simulink library "LIB_TF_G_12_StepControl"  (Simulink 8.6)
settings: Solver=ode45  StartTime=0.0  StopTime=10.0  RelTol=1e-3
PreLoadFcn:
  | if exist('tl_preloadfcn','file'), tl_preloadfcn(gcs,402); end
PostLoadFcn:
  | if exist('tl_postloadfcn','file'), tl_postloadfcn(gcs,402); end
undefined symbols (not defined in the file): ddv, u2, u3
libraries: tllib x4, LIB_TF_G_12_StepControl x1
(part 3 of 7)

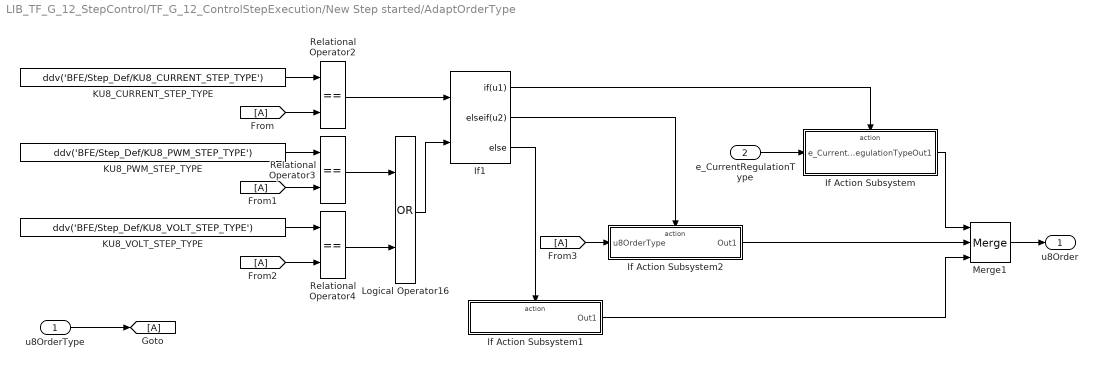
== system LIB_TF_G_12_StepControl/TF_G_12_ControlStepExecution/New Step started/AdaptOrderType ==
  u8OrderType : Inport  RequirementInfo={} %GIDa_d0932c2d_2946_4ca8_ae3e_f63aac2e144a
  e_CurrentRegulationType : Inport  RequirementInfo={} %GIDa_1019e4f9_7aa8_470e_93c0_bc7d62933626  Port=2
  If Action Subsystem : Subsystem  RequirementInfo={} %GIDa_16aa67de_e04f_4aef_8846_7bc2339db7f1  TreatAsAtomicUnit=on
  If Action Subsystem1 : Subsystem  RequirementInfo={} %GIDa_efde54be_58e1_48f4_984b_1a55cd541708  TreatAsAtomicUnit=on
  If Action Subsystem2 : Subsystem  RequirementInfo={} %GIDa_7e05d702_bec6_4133_89e3_7df1c2d817b3  TreatAsAtomicUnit=on
  If1 : If  RequirementInfo={} %GIDa_230b83ff_c373_44fd_bf0d_fc368a5a2e7f  NumInputs=2  IfExpression=u1  ElseIfExpressions=u2
  KU8_CURRENT_STEP_TYPE : Constant  RequirementInfo={} %GIDa_98379601_80fc_49bf_9245_1ac9e089f011  Value=ddv('BFE/Step_Def/KU8_CURRENT_STEP_TYPE')  OutDataTypeStr=uint8  mask(TL_Constant){data={'output',{'variable','BFE/Step_Def/KU8_CURRENT_STEP_TYPE'},'date',735951.66797598382}}
      settings: CopyFcn=if exist('tl_reset_reviewflag','file')==2,tl_reset_reviewflag(gcbh);end  DeleteFcn=if exist('delete_tlblock','file')==2,delete_tlblock(gcbh);end  NameChangeFcn=if exist('rename_tlblock','file')==2,rename_tlblock(gcbh);end  OpenFcn=if exist('tl_open_blockdlg','file')==2,tl_open_blockdlg(gcbh);else,open_system(gcbh,'parameter');end
      mask Help: eval(['if exist(''tl_online_help'',''file'') == 2, tl_online_help(''Topic'',''TL_Constant''),else, web([''jar:file:///'',matlabroot,''/help/toolbox/simulink/help.jar!/slref/' lower(get_param(gcbh,'Blocktype')) '.html''], ''-helpbrowser''),end'])
      mask Display: plot([-0.05, 1.05, NaN, -0.05, 1.05],[.01, .01, NaN, .99, .99])
  KU8_PWM_STEP_TYPE : Constant  RequirementInfo={} %GIDa_29bcd219_c5cc_40dc_ab00_ad3704692ecd  Value=ddv('BFE/Step_Def/KU8_PWM_STEP_TYPE')  OutDataTypeStr=uint8  mask(TL_Constant){data={'output',{'variable','BFE/Step_Def/KU8_PWM_STEP_TYPE'},'date',735951.66797560186}}
      settings: CopyFcn=if exist('tl_reset_reviewflag','file')==2,tl_reset_reviewflag(gcbh);end  DeleteFcn=if exist('delete_tlblock','file')==2,delete_tlblock(gcbh);end  NameChangeFcn=if exist('rename_tlblock','file')==2,rename_tlblock(gcbh);end  OpenFcn=if exist('tl_open_blockdlg','file')==2,tl_open_blockdlg(gcbh);else,open_system(gcbh,'parameter');end
      mask Help: eval(['if exist(''tl_online_help'',''file'') == 2, tl_online_help(''Topic'',''TL_Constant''),else, web([''jar:file:///'',matlabroot,''/help/toolbox/simulink/help.jar!/slref/' lower(get_param(gcbh,'Blocktype')) '.html''], ''-helpbrowser''),end'])
      mask Display: plot([-0.05, 1.05, NaN, -0.05, 1.05],[.01, .01, NaN, .99, .99])
  KU8_VOLT_STEP_TYPE : Constant  RequirementInfo={} %GIDa_f802c029_4a46_4d43_a78a_2d66bfbde5dc  Value=ddv('BFE/Step_Def/KU8_VOLT_STEP_TYPE')  OutDataTypeStr=uint8  mask(TL_Constant){data={'output',{'variable','BFE/Step_Def/KU8_VOLT_STEP_TYPE'},'date',735951.6679752199}}
      settings: CopyFcn=if exist('tl_reset_reviewflag','file')==2,tl_reset_reviewflag(gcbh);end  DeleteFcn=if exist('delete_tlblock','file')==2,delete_tlblock(gcbh);end  NameChangeFcn=if exist('rename_tlblock','file')==2,rename_tlblock(gcbh);end  OpenFcn=if exist('tl_open_blockdlg','file')==2,tl_open_blockdlg(gcbh);else,open_system(gcbh,'parameter');end
      mask Help: eval(['if exist(''tl_online_help'',''file'') == 2, tl_online_help(''Topic'',''TL_Constant''),else, web([''jar:file:///'',matlabroot,''/help/toolbox/simulink/help.jar!/slref/' lower(get_param(gcbh,'Blocktype')) '.html''], ''-helpbrowser''),end'])
      mask Display: plot([-0.05, 1.05, NaN, -0.05, 1.05],[.01, .01, NaN, .99, .99])
  Logical Operator16 : Logic  RequirementInfo={} %GIDa_b0b2f49c_87b5_4b72_83bb_2ee36afe3fae  Operator=OR  AllPortsSameDT=off  OutDataTypeStr=boolean  mask(TL_LogicalOperator){data={'date',735951.66797486111}}
      settings: DeleteFcn=if exist('delete_tlblock','file')==2,delete_tlblock(gcbh);end  NameChangeFcn=if exist('rename_tlblock','file')==2,rename_tlblock(gcbh);end  OpenFcn=if exist('tl_open_blockdlg','file')==2,tl_open_blockdlg(gcbh);else,open_system(gcbh,'parameter');end
      mask Help: eval(['if exist(''tl_online_help'',''file'') == 2, tl_online_help(''Topic'',''TL_LogicalOperator''),else, web([''jar:file:///'',matlabroot,''/help/toolbox/simulink/help.jar!/slref/' lower(get_param(gcbh,'Blocktype')) '.html''], ''-helpbrowser''),end'])
      mask Display: plot([-0.05, 1.05, NaN, -0.05, 1.05],[.01, .01, NaN, .99, .99])
  Merge1 : Merge  RequirementInfo={} %GIDa_c83b2496_f2b0_4692_be7f_77f82a802315  Inputs=3  InitialOutput=0  mask(TL_Merge){data={'output',{'name','u8NewRawOrderType'},'date',735951.66797458334}}
      settings: CopyFcn=if exist('tl_reset_reviewflag','file')==2,tl_reset_reviewflag(gcbh);end  DeleteFcn=if exist('delete_tlblock','file')==2,delete_tlblock(gcbh);end  NameChangeFcn=if exist('rename_tlblock','file')==2,rename_tlblock(gcbh);end  OpenFcn=if exist('tl_open_blockdlg','file')==2,tl_open_blockdlg(gcbh);else,open_system(gcbh,'parameter');end
      mask Help: eval(['if exist(''tl_online_help'',''file'') == 2, tl_online_help(''Topic'',''TL_Merge''),else, web([''jar:file:///'',matlabroot,''/help/toolbox/simulink/help.jar!/slref/' lower(get_param(gcbh,'Blocktype')) '.html''], ''-helpbrowser''),end'])
      mask Display: plot([-0.05, 1.05, NaN, -0.05, 1.05],[.01, .01, NaN, .99, .99])
  Relational Operator2 : RelationalOperator  RequirementInfo={} %GIDa_18ac9ebf_a7ed_4eb9_a4e9_7db870fd7569  Operator===  OutDataTypeStr=boolean  mask(TL_RelationalOperator){data={'date',735951.66797421291}}
      settings: DeleteFcn=if exist('delete_tlblock','file')==2,delete_tlblock(gcbh);end  NameChangeFcn=if exist('rename_tlblock','file')==2,rename_tlblock(gcbh);end  OpenFcn=if exist('tl_open_blockdlg','file')==2,tl_open_blockdlg(gcbh);else,open_system(gcbh,'parameter');end
      mask Help: eval(['if exist(''tl_online_help'',''file'') == 2, tl_online_help(''Topic'',''TL_RelationalOperator''),else, web([''jar:file:///'',matlabroot,''/help/toolbox/simulink/help.jar!/slref/' lower(get_param(gcbh,'Blocktype')) '.html''], ''-helpbrowser''),end'])
      mask Display: plot([-0.05, 1.05, NaN, -0.05, 1.05],[.01, .01, NaN, .99, .99])
  Relational Operator3 : RelationalOperator  RequirementInfo={} %GIDa_1f07f267_5fe9_402f_8d87_9ef376af47f7  Operator===  OutDataTypeStr=boolean  mask(TL_RelationalOperator){data={'date',735951.66797396995}}
      settings: DeleteFcn=if exist('delete_tlblock','file')==2,delete_tlblock(gcbh);end  NameChangeFcn=if exist('rename_tlblock','file')==2,rename_tlblock(gcbh);end  OpenFcn=if exist('tl_open_blockdlg','file')==2,tl_open_blockdlg(gcbh);else,open_system(gcbh,'parameter');end
      mask Help: eval(['if exist(''tl_online_help'',''file'') == 2, tl_online_help(''Topic'',''TL_RelationalOperator''),else, web([''jar:file:///'',matlabroot,''/help/toolbox/simulink/help.jar!/slref/' lower(get_param(gcbh,'Blocktype')) '.html''], ''-helpbrowser''),end'])
      mask Display: plot([-0.05, 1.05, NaN, -0.05, 1.05],[.01, .01, NaN, .99, .99])
  Relational Operator4 : RelationalOperator  RequirementInfo={} %GIDa_fd8addad_e037_4a75_aa53_445cbc8f9875  Operator===  OutDataTypeStr=boolean  mask(TL_RelationalOperator){data={'date',735951.66797372687}}
      settings: DeleteFcn=if exist('delete_tlblock','file')==2,delete_tlblock(gcbh);end  NameChangeFcn=if exist('rename_tlblock','file')==2,rename_tlblock(gcbh);end  OpenFcn=if exist('tl_open_blockdlg','file')==2,tl_open_blockdlg(gcbh);else,open_system(gcbh,'parameter');end
      mask Help: eval(['if exist(''tl_online_help'',''file'') == 2, tl_online_help(''Topic'',''TL_RelationalOperator''),else, web([''jar:file:///'',matlabroot,''/help/toolbox/simulink/help.jar!/slref/' lower(get_param(gcbh,'Blocktype')) '.html''], ''-helpbrowser''),end'])
      mask Display: plot([-0.05, 1.05, NaN, -0.05, 1.05],[.01, .01, NaN, .99, .99])
  u8Order : Outport  RequirementInfo={} %GIDa_7767866f_fef1_459c_9128_28c0971c6fc5
  wires:
  KU8_CURRENT_STEP_TYPE/1 -> Relational Operator2/1
  If1/1 -> If Action Subsystem/Action
  Relational Operator2/1 -> If1/1
  If1/3 -> If Action Subsystem1/Action
  KU8_PWM_STEP_TYPE/1 -> Relational Operator3/1
  KU8_VOLT_STEP_TYPE/1 -> Relational Operator4/1
  Relational Operator3/1 -> Logical Operator16/1
  Relational Operator4/1 -> Logical Operator16/2
  Logical Operator16/1 -> If1/2
  If1/2 -> If Action Subsystem2/Action
  u8OrderType/1 -> [A]
  [A] -> Relational Operator2/2
  [A] -> Relational Operator3/2
  [A] -> Relational Operator4/2
  [A] -> If Action Subsystem2/1(u8OrderType)
  If Action Subsystem2/1(Out1) -> Merge1/2
  If Action Subsystem1/1(Out1) -> Merge1/3
  If Action Subsystem/1(Out1) -> Merge1/1
  Merge1/1 -> u8Order/1
  e_CurrentRegulationType/1 -> If Action Subsystem/1(e_CurrentRegulationType)

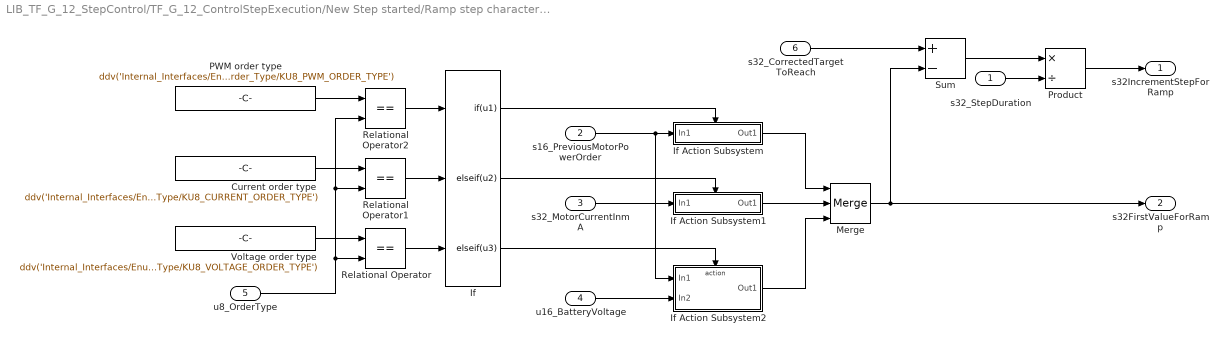
== system LIB_TF_G_12_StepControl/TF_G_12_ControlStepExecution/New Step started/Ramp step characteristics computation ==
  s32_StepDuration : Inport
  s16_PreviousMotorPowerOrder : Inport  Port=2
  s32_MotorCurrentInmA : Inport  Port=3
  u16_BatteryVoltage : Inport  Port=4
  u8_OrderType : Inport  Port=5
  s32_CorrectedTargetToReach : Inport  Port=6
  Current order type : Constant  Value=ddv('Internal_Interfaces/Enumerated_values/Step_Order_Type/KU8_CURRENT_ORDER_TYPE')  mask(TL_Constant){data={'output',{'variable','Internal_Interfaces/Enumerated_values/Step_Order_Type/KU8_CURRENT_ORDER_TYPE'},'date',735951.66797346063}}
      settings: CopyFcn=if exist('tl_reset_reviewflag','file')==2,tl_reset_reviewflag(gcbh);end  DeleteFcn=if exist('delete_tlblock','file')==2,delete_tlblock(gcbh);end  NameChangeFcn=if exist('rename_tlblock','file')==2,rename_tlblock(gcbh);end  OpenFcn=if exist('tl_open_blockdlg','file')==2,tl_open_blockdlg(gcbh);else,open_system(gcbh,'parameter');end
      mask Help: eval(['if exist(''tl_online_help'',''file'') == 2, tl_online_help(''Topic'',''TL_Constant''),else, web([''jar:file:///'',matlabroot,''/help/toolbox/simulink/help.jar!/slref/' lower(get_param(gcbh,'Blocktype')) '.html''], ''-helpbrowser''),end'])
      mask Display: plot([-0.05, 1.05, NaN, -0.05, 1.05],[.01, .01, NaN, .99, .99])
  If : If  NumInputs=3  IfExpression=u1  ElseIfExpressions=u2,u3  ShowElse=off
  If Action Subsystem : Subsystem  TreatAsAtomicUnit=on
  If Action Subsystem1 : Subsystem  TreatAsAtomicUnit=on
  If Action Subsystem2 : Subsystem  TreatAsAtomicUnit=on
  Merge : Merge  Inputs=3  InitialOutput=0  mask(TL_Merge){data={'output',{'name','s32FirstValueForRampStep'},'date',735951.66796866897}}
      settings: CopyFcn=if exist('tl_reset_reviewflag','file')==2,tl_reset_reviewflag(gcbh);end  DeleteFcn=if exist('delete_tlblock','file')==2,delete_tlblock(gcbh);end  NameChangeFcn=if exist('rename_tlblock','file')==2,rename_tlblock(gcbh);end  OpenFcn=if exist('tl_open_blockdlg','file')==2,tl_open_blockdlg(gcbh);else,open_system(gcbh,'parameter');end
      mask Help: eval(['if exist(''tl_online_help'',''file'') == 2, tl_online_help(''Topic'',''TL_Merge''),else, web([''jar:file:///'',matlabroot,''/help/toolbox/simulink/help.jar!/slref/' lower(get_param(gcbh,'Blocktype')) '.html''], ''-helpbrowser''),end'])
      mask Display: plot([-0.05, 1.05, NaN, -0.05, 1.05],[.01, .01, NaN, .99, .99])
  PWM order type : Constant  Value=ddv('Internal_Interfaces/Enumerated_values/Step_Order_Type/KU8_PWM_ORDER_TYPE')  mask(TL_Constant){data={'output',{'variable','Internal_Interfaces/Enumerated_values/Step_Order_Type/KU8_PWM_ORDER_TYPE'},'date',735951.66796828702}}
      settings: CopyFcn=if exist('tl_reset_reviewflag','file')==2,tl_reset_reviewflag(gcbh);end  DeleteFcn=if exist('delete_tlblock','file')==2,delete_tlblock(gcbh);end  NameChangeFcn=if exist('rename_tlblock','file')==2,rename_tlblock(gcbh);end  OpenFcn=if exist('tl_open_blockdlg','file')==2,tl_open_blockdlg(gcbh);else,open_system(gcbh,'parameter');end
      mask Help: eval(['if exist(''tl_online_help'',''file'') == 2, tl_online_help(''Topic'',''TL_Constant''),else, web([''jar:file:///'',matlabroot,''/help/toolbox/simulink/help.jar!/slref/' lower(get_param(gcbh,'Blocktype')) '.html''], ''-helpbrowser''),end'])
      mask Display: plot([-0.05, 1.05, NaN, -0.05, 1.05],[.01, .01, NaN, .99, .99])
  Product : Product  Inputs=*/  OutDataTypeStr=int32  RndMeth=Zero  mask(TL_Product){data={'output',{'name','s32IncrementForRampStep','type','Int32'},'exceptionhandling',0,'date',735951.66796789353}}
      settings: CopyFcn=if exist('tl_reset_reviewflag','file')==2,tl_reset_reviewflag(gcbh);end  DeleteFcn=if exist('delete_tlblock','file')==2,delete_tlblock(gcbh);end  NameChangeFcn=if exist('rename_tlblock','file')==2,rename_tlblock(gcbh);end  OpenFcn=if exist('tl_open_blockdlg','file')==2,tl_open_blockdlg(gcbh);else,open_system(gcbh,'parameter');end
      mask Help: eval(['if exist(''tl_online_help'',''file'') == 2, tl_online_help(''Topic'',''TL_Product''),else, web([''jar:file:///'',matlabroot,''/help/toolbox/simulink/help.jar!/slref/' lower(get_param(gcbh,'Blocktype')) '.html''], ''-helpbrowser''),end'])
      mask Display: plot([-0.05, 1.05, NaN, -0.05, 1.05],[.01, .01, NaN, .99, .99])
  Relational Operator : RelationalOperator  Operator===  OutDataTypeStr=boolean  mask(TL_RelationalOperator){data={'date',735951.66796754627}}
      settings: DeleteFcn=if exist('delete_tlblock','file')==2,delete_tlblock(gcbh);end  NameChangeFcn=if exist('rename_tlblock','file')==2,rename_tlblock(gcbh);end  OpenFcn=if exist('tl_open_blockdlg','file')==2,tl_open_blockdlg(gcbh);else,open_system(gcbh,'parameter');end
      mask Help: eval(['if exist(''tl_online_help'',''file'') == 2, tl_online_help(''Topic'',''TL_RelationalOperator''),else, web([''jar:file:///'',matlabroot,''/help/toolbox/simulink/help.jar!/slref/' lower(get_param(gcbh,'Blocktype')) '.html''], ''-helpbrowser''),end'])
      mask Display: plot([-0.05, 1.05, NaN, -0.05, 1.05],[.01, .01, NaN, .99, .99])
  Relational Operator1 : RelationalOperator  Operator===  OutDataTypeStr=boolean  mask(TL_RelationalOperator){data={'date',735951.66796729167}}
      settings: DeleteFcn=if exist('delete_tlblock','file')==2,delete_tlblock(gcbh);end  NameChangeFcn=if exist('rename_tlblock','file')==2,rename_tlblock(gcbh);end  OpenFcn=if exist('tl_open_blockdlg','file')==2,tl_open_blockdlg(gcbh);else,open_system(gcbh,'parameter');end
      mask Help: eval(['if exist(''tl_online_help'',''file'') == 2, tl_online_help(''Topic'',''TL_RelationalOperator''),else, web([''jar:file:///'',matlabroot,''/help/toolbox/simulink/help.jar!/slref/' lower(get_param(gcbh,'Blocktype')) '.html''], ''-helpbrowser''),end'])
      mask Display: plot([-0.05, 1.05, NaN, -0.05, 1.05],[.01, .01, NaN, .99, .99])
  Relational Operator2 : RelationalOperator  Operator===  OutDataTypeStr=boolean  mask(TL_RelationalOperator){data={'date',735951.66796704859}}
      settings: DeleteFcn=if exist('delete_tlblock','file')==2,delete_tlblock(gcbh);end  NameChangeFcn=if exist('rename_tlblock','file')==2,rename_tlblock(gcbh);end  OpenFcn=if exist('tl_open_blockdlg','file')==2,tl_open_blockdlg(gcbh);else,open_system(gcbh,'parameter');end
      mask Help: eval(['if exist(''tl_online_help'',''file'') == 2, tl_online_help(''Topic'',''TL_RelationalOperator''),else, web([''jar:file:///'',matlabroot,''/help/toolbox/simulink/help.jar!/slref/' lower(get_param(gcbh,'Blocktype')) '.html''], ''-helpbrowser''),end'])
      mask Display: plot([-0.05, 1.05, NaN, -0.05, 1.05],[.01, .01, NaN, .99, .99])
  Sum : Sum  Inputs=+-  mask(TL_Sum){data={'output',{'type','Int32'},'date',735951.66796678246}}
      settings: CopyFcn=if exist('tl_reset_reviewflag','file')==2,tl_reset_reviewflag(gcbh);end  DeleteFcn=if exist('delete_tlblock','file')==2,delete_tlblock(gcbh);end  NameChangeFcn=if exist('rename_tlblock','file')==2,rename_tlblock(gcbh);end  OpenFcn=if exist('tl_open_blockdlg','file')==2,tl_open_blockdlg(gcbh);else,open_system(gcbh,'parameter');end
      mask Help: eval(['if exist(''tl_online_help'',''file'') == 2, tl_online_help(''Topic'',''TL_Sum''),else, web([''jar:file:///'',matlabroot,''/help/toolbox/simulink/help.jar!/slref/' lower(get_param(gcbh,'Blocktype')) '.html''], ''-helpbrowser''),end'])
      mask Display: plot([-0.05, 1.05, NaN, -0.05, 1.05],[.01, .01, NaN, .99, .99])
  Voltage order type : Constant  Value=ddv('Internal_Interfaces/Enumerated_values/Step_Order_Type/KU8_VOLTAGE_ORDER_TYPE')  mask(TL_Constant){data={'output',{'variable','Internal_Interfaces/Enumerated_values/Step_Order_Type/KU8_VOLTAGE_ORDER_TYPE'},'date',735951.6679664352}}
      settings: CopyFcn=if exist('tl_reset_reviewflag','file')==2,tl_reset_reviewflag(gcbh);end  DeleteFcn=if exist('delete_tlblock','file')==2,delete_tlblock(gcbh);end  NameChangeFcn=if exist('rename_tlblock','file')==2,rename_tlblock(gcbh);end  OpenFcn=if exist('tl_open_blockdlg','file')==2,tl_open_blockdlg(gcbh);else,open_system(gcbh,'parameter');end
      mask Help: eval(['if exist(''tl_online_help'',''file'') == 2, tl_online_help(''Topic'',''TL_Constant''),else, web([''jar:file:///'',matlabroot,''/help/toolbox/simulink/help.jar!/slref/' lower(get_param(gcbh,'Blocktype')) '.html''], ''-helpbrowser''),end'])
      mask Display: plot([-0.05, 1.05, NaN, -0.05, 1.05],[.01, .01, NaN, .99, .99])
  s32IncrementStepForRamp : Outport
  s32FirstValueForRamp : Outport  Port=2
  wires:
  Voltage order type/1 -> Relational Operator/1
  Current order type/1 -> Relational Operator1/1
  PWM order type/1 -> Relational Operator2/1
  u8_OrderType/1 -> Relational Operator/2, Relational Operator1/2, Relational Operator2/2
  Relational Operator2/1 -> If/1
  Relational Operator1/1 -> If/2
  Relational Operator/1 -> If/3
  If/1 -> If Action Subsystem/Action
  s16_PreviousMotorPowerOrder/1 -> If Action Subsystem/1(In1), If Action Subsystem2/1(In1)
  s32_MotorCurrentInmA/1 -> If Action Subsystem1/1(In1)
  If/2 -> If Action Subsystem1/Action
  If/3 -> If Action Subsystem2/Action
  u16_BatteryVoltage/1 -> If Action Subsystem2/2(In2)
  If Action Subsystem/1(Out1) -> Merge/1
  If Action Subsystem1/1(Out1) -> Merge/2
  If Action Subsystem2/1(Out1) -> Merge/3
  Merge/1 -> s32FirstValueForRamp/1, Sum/2
  s32_CorrectedTargetToReach/1 -> Sum/1
  Sum/1 -> Product/1
  Product/1 -> s32IncrementStepForRamp/1
  s32_StepDuration/1 -> Product/2

== system LIB_TF_G_12_StepControl/TF_G_12_ControlStepExecution/New Step started/RescaleStepDuration ==
  u16Time : Inport  RequirementInfo={} %GIDa_7ed774dc_7342_452f_a0c9_75f50665b992
  Constant : Constant  RequirementInfo={} %GIDa_5b829873_6cd2_402b_a0cb_d7ea2bf2d5e1  Value=ddv('Sampling_Freq/KUS_MOTOR_PERIOD')  OutDataTypeStr=uint16  mask(TL_Constant){data={'output',{'variable','Sampling_Freq/KUS_MOTOR_PERIOD'},'date',735951.66796605324}}
      settings: CopyFcn=if exist('tl_reset_reviewflag','file')==2,tl_reset_reviewflag(gcbh);end  DeleteFcn=if exist('delete_tlblock','file')==2,delete_tlblock(gcbh);end  NameChangeFcn=if exist('rename_tlblock','file')==2,rename_tlblock(gcbh);end  OpenFcn=if exist('tl_open_blockdlg','file')==2,tl_open_blockdlg(gcbh);else,open_system(gcbh,'parameter');end
      mask Help: eval(['if exist(''tl_online_help'',''file'') == 2, tl_online_help(''Topic'',''TL_Constant''),else, web([''jar:file:///'',matlabroot,''/help/toolbox/simulink/help.jar!/slref/' lower(get_param(gcbh,'Blocktype')) '.html''], ''-helpbrowser''),end'])
      mask Display: plot([-0.05, 1.05, NaN, -0.05, 1.05],[.01, .01, NaN, .99, .99])
  Constant1 : Constant  RequirementInfo={} %GIDa_4a578cf0_e6d7_4c27_85f7_4ca2cc919af8  Value=ddv('Sampling_Freq/KUS_STEP_SELECTION_PERIOD')  OutDataTypeStr=uint16  mask(TL_Constant){data={'output',{'variable','Sampling_Freq/KUS_STEP_SELECTION_PERIOD'},'date',735951.66796567128}}
      settings: CopyFcn=if exist('tl_reset_reviewflag','file')==2,tl_reset_reviewflag(gcbh);end  DeleteFcn=if exist('delete_tlblock','file')==2,delete_tlblock(gcbh);end  NameChangeFcn=if exist('rename_tlblock','file')==2,rename_tlblock(gcbh);end  OpenFcn=if exist('tl_open_blockdlg','file')==2,tl_open_blockdlg(gcbh);else,open_system(gcbh,'parameter');end
      mask Help: eval(['if exist(''tl_online_help'',''file'') == 2, tl_online_help(''Topic'',''TL_Constant''),else, web([''jar:file:///'',matlabroot,''/help/toolbox/simulink/help.jar!/slref/' lower(get_param(gcbh,'Blocktype')) '.html''], ''-helpbrowser''),end'])
      mask Display: plot([-0.05, 1.05, NaN, -0.05, 1.05],[.01, .01, NaN, .99, .99])
  Divide : Product  RequirementInfo={} %GIDa_6bac047a_3eab_476b_8a0a_99d834524f2c  Inputs=*/  OutDataTypeStr=uint16  mask(TL_Product){data={'output',{'type','UInt16'},'date',735951.66796528932}}
      settings: CopyFcn=if exist('tl_reset_reviewflag','file')==2,tl_reset_reviewflag(gcbh);end  DeleteFcn=if exist('delete_tlblock','file')==2,delete_tlblock(gcbh);end  NameChangeFcn=if exist('rename_tlblock','file')==2,rename_tlblock(gcbh);end  OpenFcn=if exist('tl_open_blockdlg','file')==2,tl_open_blockdlg(gcbh);else,open_system(gcbh,'parameter');end
      mask Help: eval(['if exist(''tl_online_help'',''file'') == 2, tl_online_help(''Topic'',''TL_Product''),else, web([''jar:file:///'',matlabroot,''/help/toolbox/simulink/help.jar!/slref/' lower(get_param(gcbh,'Blocktype')) '.html''], ''-helpbrowser''),end'])
      mask Display: plot([-0.05, 1.05, NaN, -0.05, 1.05],[.01, .01, NaN, .99, .99])
  Product : Product  RequirementInfo={} %GIDa_2b507d9b_40a7_451c_a7a8_cd6f5fc7de83  OutDataTypeStr=int32  SaturateOnIntegerOverflow=on  RndMeth=Zero  mask(TL_Product){data={'output',{'name','s32TimeHighResolution','type','Int32','checkmin',1,'checkmax',1},'date',735951.66796490736}}
      settings: CopyFcn=if exist('tl_reset_reviewflag','file')==2,tl_reset_reviewflag(gcbh);end  DeleteFcn=if exist('delete_tlblock','file')==2,delete_tlblock(gcbh);end  NameChangeFcn=if exist('rename_tlblock','file')==2,rename_tlblock(gcbh);end  OpenFcn=if exist('tl_open_blockdlg','file')==2,tl_open_blockdlg(gcbh);else,open_system(gcbh,'parameter');end
      mask Help: eval(['if exist(''tl_online_help'',''file'') == 2, tl_online_help(''Topic'',''TL_Product''),else, web([''jar:file:///'',matlabroot,''/help/toolbox/simulink/help.jar!/slref/' lower(get_param(gcbh,'Blocktype')) '.html''], ''-helpbrowser''),end'])
      mask Display: plot([-0.05, 1.05, NaN, -0.05, 1.05],[.01, .01, NaN, .99, .99])
  s32TimeHighResolution : Outport  RequirementInfo={} %GIDa_7022b762_a0d5_4516_ba29_420e6b8c6fab
  wires:
  Divide/1 -> Product/1
  Constant/1 -> Divide/2
  Constant1/1 -> Divide/1
  Product/1 -> s32TimeHighResolution/1
  u16Time/1 -> Product/2

== system LIB_TF_G_12_StepControl/TF_G_12_ManageEndingStep/Step execution in progress/ManageAdaptiveCurrentInterruptionPoint (Comfort Belt Functions) ==
  u8AdaptiveCurrentLimitation : Inport  RequirementInfo={} %GIDa_cf26c4a4_ab72_4e01_b0f8_8861d02ea64d
  u32MotorCurrent : Inport  RequirementInfo={} %GIDa_0406aca6_3c48_472e_97d4_b3729755944d  Port=2
  u16Temperature : Inport  RequirementInfo={} %GIDa_178059e8_7d65_4de1_9690_4cb4c0d47300  Port=3
  Constant2 : Constant  RequirementInfo={} %GIDa_a9cdef41_d9d0_4a8e_913e_e30434a32e14  SampleTime=-1  mask(TL_Constant){data={'output',{'variable','BFE_Config_PreProc/BFE_CFG_OPT_ADAPT_CURRENT'},'date',735951.66848431714}}
      settings: CopyFcn=if exist('tl_reset_reviewflag','file')==2,tl_reset_reviewflag(gcbh);end  DeleteFcn=if exist('delete_tlblock','file')==2,delete_tlblock(gcbh);end  NameChangeFcn=if exist('rename_tlblock','file')==2,rename_tlblock(gcbh);end  OpenFcn=if exist('tl_open_blockdlg','file')==2,tl_open_blockdlg(gcbh);else,open_system(gcbh,'parameter');end
      mask Help: eval(['if exist(''tl_online_help'',''file'') == 2, tl_online_help(''Topic'',''TL_Constant''),else, web([''jar:file:///'',matlabroot,''/help/toolbox/simulink/help.jar!/slref/' lower(get_param(gcbh,'Blocktype')) '.html''], ''-helpbrowser''),end'])
      mask Display: plot([-0.05, 1.05, NaN, -0.05, 1.05],[.01, .01, NaN, .99, .99])
  Current Int Point Opt Activated : Subsystem  RequirementInfo={} %GIDa_8be4b952_f9f7_4f2b_b897_8f333789c9df  TreatAsAtomicUnit=on
  Current Int Point Opt Deactivated : Subsystem  RequirementInfo={} %GIDa_df64a73f_f3f0_40be_a0eb_a00783f34347  TreatAsAtomicUnit=on
  Merge : Merge  Description=bTriggOffEvent :  RequirementInfo={} %GIDa_869a9126_8289_4d79_9e68_a6566189ca3d  InitialOutput=1  mask(TL_Merge){data={'comment',{'text',['bTriggOffEvent :']},'output',{'name','bCurrentInterruptionPointEvent'},'date',735951.66847956018}}
      settings: CopyFcn=if exist('tl_reset_reviewflag','file')==2,tl_reset_reviewflag(gcbh);end  DeleteFcn=if exist('delete_tlblock','file')==2,delete_tlblock(gcbh);end  NameChangeFcn=if exist('rename_tlblock','file')==2,rename_tlblock(gcbh);end  OpenFcn=if exist('tl_open_blockdlg','file')==2,tl_open_blockdlg(gcbh);else,open_system(gcbh,'parameter');end
      mask Help: eval(['if exist(''tl_online_help'',''file'') == 2, tl_online_help(''Topic'',''TL_Merge''),else, web([''jar:file:///'',matlabroot,''/help/toolbox/simulink/help.jar!/slref/' lower(get_param(gcbh,'Blocktype')) '.html''], ''-helpbrowser''),end'])
      mask Display: plot([-0.05, 1.05, NaN, -0.05, 1.05],[.01, .01, NaN, .99, .99])
  Preprocessor IF : If  RequirementInfo={} %GIDa_f2532fbd_a45e_4a30_b23b_b51771a5e750  IfExpression=u1  mask(TL_PreProcessorIf){data={'mode',2,'date',735951.66847923608}}
      settings: DeleteFcn=if exist('delete_tlblock','file')==2,delete_tlblock(gcbh);end  NameChangeFcn=if exist('rename_tlblock','file')==2,rename_tlblock(gcbh);end  OpenFcn=if exist('tl_open_blockdlg','file')==2,tl_open_blockdlg(gcbh);else,open_system(gcbh,'parameter');end
      mask Help: eval(['if exist(''tl_online_help'',''file'') == 2, tl_online_help(''Topic'',''TL_PreProcessorIf''),else, web([''jar:file:///'',matlabroot,''/help/toolbox/simulink/help.jar!/slref/' lower(get_param(gcbh,'Blocktype')) '.html''], ''-helpbrowser''),end'])
      mask Display:
      | plot([-0.05, 1.05, NaN, -0.05, 1.05],[.01, .01, NaN, .99, .99])
      | 
      | port_label('input', 1, 'u1')
      | port_label('output',1,'#ifdef u1');
      | port_label('output',2,'#else');
  bInterruptStep : Outport  RequirementInfo={} %GIDa_57554a0d_af87_47fa_85ff_f29dcf962e81
  wires:
  Preprocessor IF/1 -> Current Int Point Opt Activated/Action
  Preprocessor IF/2 -> Current Int Point Opt Deactivated/Action
  Current Int Point Opt Deactivated/1(bInterruptStep) -> Merge/1
  Constant2/1 -> Preprocessor IF/1
  Merge/1 -> bInterruptStep/1
  Current Int Point Opt Activated/1(bInterruptStep) -> Merge/2
  u8AdaptiveCurrentLimitation/1 -> Current Int Point Opt Activated/1(u8AdaptiveCurrentLimitation)
  u32MotorCurrent/1 -> Current Int Point Opt Activated/2(u32MotorCurrent)
  u16Temperature/1 -> Current Int Point Opt Activated/3(u16Temperature)

== system LIB_TF_G_12_StepControl/TF_G_12_ManageEndingStep/Step execution in progress/ManageBeltBlocked (HES sensors) ==
  bBeltBlockedControlled : Inport  RequirementInfo={} %GIDa_b3b829c7_707e_4393_b518_07c2361378f2
  s32BeltSpeed : Inport  RequirementInfo={} %GIDa_b465a0f2_96a3_4d05_9aec_c0287b1f40e7  Port=2
  Belt Blocked Opt Activated : Subsystem  RequirementInfo={} %GIDa_4fe18e08_833a_4167_87cd_2334fd4970d3  TreatAsAtomicUnit=on
  Belt Blocked Opt Deactivated : Subsystem  RequirementInfo={} %GIDa_62be95f4_4e3a_4669_9689_11d27973e356  TreatAsAtomicUnit=on
  Constant : Constant  RequirementInfo={} %GIDa_bb502461_7a2b_44ab_8b1d_ba4b923b2750  SampleTime=-1  mask(TL_Constant){data={'output',{'variable','BFE_Config_PreProc/BFE_CFG_OPT_BELT_BLOCKED_HES'},'date',735951.66847781255}}
      settings: CopyFcn=if exist('tl_reset_reviewflag','file')==2,tl_reset_reviewflag(gcbh);end  DeleteFcn=if exist('delete_tlblock','file')==2,delete_tlblock(gcbh);end  NameChangeFcn=if exist('rename_tlblock','file')==2,rename_tlblock(gcbh);end  OpenFcn=if exist('tl_open_blockdlg','file')==2,tl_open_blockdlg(gcbh);else,open_system(gcbh,'parameter');end
      mask Help: eval(['if exist(''tl_online_help'',''file'') == 2, tl_online_help(''Topic'',''TL_Constant''),else, web([''jar:file:///'',matlabroot,''/help/toolbox/simulink/help.jar!/slref/' lower(get_param(gcbh,'Blocktype')) '.html''], ''-helpbrowser''),end'])
      mask Display: plot([-0.05, 1.05, NaN, -0.05, 1.05],[.01, .01, NaN, .99, .99])
  Merge : Merge  Description=bTriggOffEvent :  RequirementInfo={} %GIDa_907c82db_0dea_4729_bb50_e876116e174f  InitialOutput=1  mask(TL_Merge){data={'comment',{'text',['bTriggOffEvent :']},'output',{'name','bBeltBlockedEvent'},'date',735951.66847743059}}
      settings: CopyFcn=if exist('tl_reset_reviewflag','file')==2,tl_reset_reviewflag(gcbh);end  DeleteFcn=if exist('delete_tlblock','file')==2,delete_tlblock(gcbh);end  NameChangeFcn=if exist('rename_tlblock','file')==2,rename_tlblock(gcbh);end  OpenFcn=if exist('tl_open_blockdlg','file')==2,tl_open_blockdlg(gcbh);else,open_system(gcbh,'parameter');end
      mask Help: eval(['if exist(''tl_online_help'',''file'') == 2, tl_online_help(''Topic'',''TL_Merge''),else, web([''jar:file:///'',matlabroot,''/help/toolbox/simulink/help.jar!/slref/' lower(get_param(gcbh,'Blocktype')) '.html''], ''-helpbrowser''),end'])
      mask Display: plot([-0.05, 1.05, NaN, -0.05, 1.05],[.01, .01, NaN, .99, .99])
  Preprocessor IF : If  RequirementInfo={} %GIDa_fa2c6d5d_92b0_4b3b_be60_0bc11928834f  IfExpression=u1  mask(TL_PreProcessorIf){data={'mode',2,'date',735951.66847711802}}
      settings: DeleteFcn=if exist('delete_tlblock','file')==2,delete_tlblock(gcbh);end  NameChangeFcn=if exist('rename_tlblock','file')==2,rename_tlblock(gcbh);end  OpenFcn=if exist('tl_open_blockdlg','file')==2,tl_open_blockdlg(gcbh);else,open_system(gcbh,'parameter');end
      mask Help: eval(['if exist(''tl_online_help'',''file'') == 2, tl_online_help(''Topic'',''TL_PreProcessorIf''),else, web([''jar:file:///'',matlabroot,''/help/toolbox/simulink/help.jar!/slref/' lower(get_param(gcbh,'Blocktype')) '.html''], ''-helpbrowser''),end'])
      mask Display:
      | plot([-0.05, 1.05, NaN, -0.05, 1.05],[.01, .01, NaN, .99, .99])
      | 
      | port_label('input', 1, 'u1')
      | port_label('output',1,'#ifdef u1');
      | port_label('output',2,'#else');
  bInterruptStep : Outport  RequirementInfo={} %GIDa_4c6b3faf_719e_4f75_8b44_68731f30800a
  wires:
  Constant/1 -> Preprocessor IF/1
  s32BeltSpeed/1 -> Belt Blocked Opt Activated/2(s32BeltSpeed)
  bBeltBlockedControlled/1 -> Belt Blocked Opt Activated/1(bBeltBlockedControlled)
  Belt Blocked Opt Deactivated/1(bInterruptStep) -> Merge/1
  Belt Blocked Opt Activated/1(bInterruptStep) -> Merge/2
  Preprocessor IF/2 -> Belt Blocked Opt Deactivated/Action
  Preprocessor IF/1 -> Belt Blocked Opt Activated/Action
  Merge/1 -> bInterruptStep/1

== system LIB_TF_G_12_StepControl/TF_G_12_ManageEndingStep/Step execution in progress/ManageBeltMvtDetection (HES sensors) ==
  bBeltMvtDetection : Inport  RequirementInfo={} %GIDa_9c632158_4892_474c_99bd_0089793e5e05
  s32BeltSpeed : Inport  RequirementInfo={} %GIDa_db0a6ef8_ed18_42c7_bcd0_065e5905be29  Port=2
  Belt Mvt Detect Opt Activated : Subsystem  RequirementInfo={} %GIDa_781052d0_5c6a_4d3e_beae_ba59dc611bd6  TreatAsAtomicUnit=on
  Belt Mvt Detect Opt Deactivated : Subsystem  RequirementInfo={} %GIDa_adc98f89_75e9_457e_aeea_c74dc8fdc5c1  TreatAsAtomicUnit=on
  Constant : Constant  RequirementInfo={} %GIDa_5ba85715_6fd0_4828_962c_79e10967d540  SampleTime=-1  mask(TL_Constant){data={'output',{'variable','BFE_Config_PreProc/BFE_CFG_OPT_BELT_MVT_DETECT'},'date',735951.66847568285}}
      settings: CopyFcn=if exist('tl_reset_reviewflag','file')==2,tl_reset_reviewflag(gcbh);end  DeleteFcn=if exist('delete_tlblock','file')==2,delete_tlblock(gcbh);end  NameChangeFcn=if exist('rename_tlblock','file')==2,rename_tlblock(gcbh);end  OpenFcn=if exist('tl_open_blockdlg','file')==2,tl_open_blockdlg(gcbh);else,open_system(gcbh,'parameter');end
      mask Help: eval(['if exist(''tl_online_help'',''file'') == 2, tl_online_help(''Topic'',''TL_Constant''),else, web([''jar:file:///'',matlabroot,''/help/toolbox/simulink/help.jar!/slref/' lower(get_param(gcbh,'Blocktype')) '.html''], ''-helpbrowser''),end'])
      mask Display: plot([-0.05, 1.05, NaN, -0.05, 1.05],[.01, .01, NaN, .99, .99])
  Merge : Merge  Description=bTriggOffEvent :  RequirementInfo={} %GIDa_9b9442d8_ebe3_4ca4_bc8d_9653467c24ef  InitialOutput=1  mask(TL_Merge){data={'comment',{'text',['bTriggOffEvent :']},'output',{'name','bBeltMvtEvent'},'date',735951.66847530089}}
      settings: CopyFcn=if exist('tl_reset_reviewflag','file')==2,tl_reset_reviewflag(gcbh);end  DeleteFcn=if exist('delete_tlblock','file')==2,delete_tlblock(gcbh);end  NameChangeFcn=if exist('rename_tlblock','file')==2,rename_tlblock(gcbh);end  OpenFcn=if exist('tl_open_blockdlg','file')==2,tl_open_blockdlg(gcbh);else,open_system(gcbh,'parameter');end
      mask Help: eval(['if exist(''tl_online_help'',''file'') == 2, tl_online_help(''Topic'',''TL_Merge''),else, web([''jar:file:///'',matlabroot,''/help/toolbox/simulink/help.jar!/slref/' lower(get_param(gcbh,'Blocktype')) '.html''], ''-helpbrowser''),end'])
      mask Display: plot([-0.05, 1.05, NaN, -0.05, 1.05],[.01, .01, NaN, .99, .99])
  Preprocessor IF : If  RequirementInfo={} %GIDa_69cec197_646f_4cd8_9662_70000fbade2e  IfExpression=u1  mask(TL_PreProcessorIf){data={'mode',2,'date',735951.66847498843}}
      settings: DeleteFcn=if exist('delete_tlblock','file')==2,delete_tlblock(gcbh);end  NameChangeFcn=if exist('rename_tlblock','file')==2,rename_tlblock(gcbh);end  OpenFcn=if exist('tl_open_blockdlg','file')==2,tl_open_blockdlg(gcbh);else,open_system(gcbh,'parameter');end
      mask Help: eval(['if exist(''tl_online_help'',''file'') == 2, tl_online_help(''Topic'',''TL_PreProcessorIf''),else, web([''jar:file:///'',matlabroot,''/help/toolbox/simulink/help.jar!/slref/' lower(get_param(gcbh,'Blocktype')) '.html''], ''-helpbrowser''),end'])
      mask Display:
      | plot([-0.05, 1.05, NaN, -0.05, 1.05],[.01, .01, NaN, .99, .99])
      | 
      | port_label('input', 1, 'u1')
      | port_label('output',1,'#ifdef u1');
      | port_label('output',2,'#else');
  bInterruptStep : Outport  RequirementInfo={} %GIDa_36cf7132_7507_4ea2_94db_68efc3a553eb
  wires:
  Merge/1 -> bInterruptStep/1
  Preprocessor IF/1 -> Belt Mvt Detect Opt Activated/Action
  Preprocessor IF/2 -> Belt Mvt Detect Opt Deactivated/Action
  Belt Mvt Detect Opt Activated/1(bInterruptStep) -> Merge/2
  Belt Mvt Detect Opt Deactivated/1(bInterruptStep) -> Merge/1
  bBeltMvtDetection/1 -> Belt Mvt Detect Opt Activated/1(bBeltMvtDetection)
  s32BeltSpeed/1 -> Belt Mvt Detect Opt Activated/2(s32BeltSpeed)
  Constant/1 -> Preprocessor IF/1

== system LIB_TF_G_12_StepControl/TF_G_12_ManageEndingStep/Step execution in progress/ManageBeltPayOutAbortion ==
  bBeltPayOutAbortion2 : Inport  RequirementInfo={} %GIDa_7244bcd6_2a9a_48e3_a6aa_ea6abb1d027d
  bBeltPayOutAbortion1 : Inport  RequirementInfo={} %GIDa_194d2a71_0316_4b8b_9113_3d3f050cfc9c  Port=2
  u16BeltPayOutFiltered_mm : Inport  RequirementInfo={} %GIDa_ed79c04c_a1ef_40a3_9f1f_707898804cb5  Port=3
  Belt Payout Abortion Opt Activated : Subsystem  RequirementInfo={} %GIDa_1e8e8f68_dbe6_45a2_b8f3_7dbe832e4a58  TreatAsAtomicUnit=on
  Belt Payout Abortion Opt Deactivated : Subsystem  RequirementInfo={} %GIDa_e655cf51_2291_491f_aaed_19e917c7151e  TreatAsAtomicUnit=on
  Constant : Constant  RequirementInfo={} %GIDa_e9812538_195c_476c_805c_23559fab0270  SampleTime=-1  mask(TL_Constant){data={'output',{'variable','BFE_Config_PreProc/BFE_CFG_OPT_BELT_PAYOUT_ABORTION'},'date',735951.66847211809}}
      settings: CopyFcn=if exist('tl_reset_reviewflag','file')==2,tl_reset_reviewflag(gcbh);end  DeleteFcn=if exist('delete_tlblock','file')==2,delete_tlblock(gcbh);end  NameChangeFcn=if exist('rename_tlblock','file')==2,rename_tlblock(gcbh);end  OpenFcn=if exist('tl_open_blockdlg','file')==2,tl_open_blockdlg(gcbh);else,open_system(gcbh,'parameter');end
      mask Help: eval(['if exist(''tl_online_help'',''file'') == 2, tl_online_help(''Topic'',''TL_Constant''),else, web([''jar:file:///'',matlabroot,''/help/toolbox/simulink/help.jar!/slref/' lower(get_param(gcbh,'Blocktype')) '.html''], ''-helpbrowser''),end'])
      mask Display: plot([-0.05, 1.05, NaN, -0.05, 1.05],[.01, .01, NaN, .99, .99])
  Merge : Merge  Description=bTriggOffEvent :  RequirementInfo={} %GIDa_04d23865_db84_4148_9d29_a05a1e9bcf70  InitialOutput=1  mask(TL_Merge){data={'comment',{'text',['bTriggOffEvent :']},'output',{'name','bBeltPayoutEvent'},'date',735951.6684717593}}
      settings: CopyFcn=if exist('tl_reset_reviewflag','file')==2,tl_reset_reviewflag(gcbh);end  DeleteFcn=if exist('delete_tlblock','file')==2,delete_tlblock(gcbh);end  NameChangeFcn=if exist('rename_tlblock','file')==2,rename_tlblock(gcbh);end  OpenFcn=if exist('tl_open_blockdlg','file')==2,tl_open_blockdlg(gcbh);else,open_system(gcbh,'parameter');end
      mask Help: eval(['if exist(''tl_online_help'',''file'') == 2, tl_online_help(''Topic'',''TL_Merge''),else, web([''jar:file:///'',matlabroot,''/help/toolbox/simulink/help.jar!/slref/' lower(get_param(gcbh,'Blocktype')) '.html''], ''-helpbrowser''),end'])
      mask Display: plot([-0.05, 1.05, NaN, -0.05, 1.05],[.01, .01, NaN, .99, .99])
  Preprocessor IF : If  RequirementInfo={} %GIDa_423d203c_34e9_4013_9845_af154f11e5ed  IfExpression=u1  mask(TL_PreProcessorIf){data={'mode',2,'date',735951.6684714352}}
      settings: DeleteFcn=if exist('delete_tlblock','file')==2,delete_tlblock(gcbh);end  NameChangeFcn=if exist('rename_tlblock','file')==2,rename_tlblock(gcbh);end  OpenFcn=if exist('tl_open_blockdlg','file')==2,tl_open_blockdlg(gcbh);else,open_system(gcbh,'parameter');end
      mask Help: eval(['if exist(''tl_online_help'',''file'') == 2, tl_online_help(''Topic'',''TL_PreProcessorIf''),else, web([''jar:file:///'',matlabroot,''/help/toolbox/simulink/help.jar!/slref/' lower(get_param(gcbh,'Blocktype')) '.html''], ''-helpbrowser''),end'])
      mask Display:
      | plot([-0.05, 1.05, NaN, -0.05, 1.05],[.01, .01, NaN, .99, .99])
      | 
      | port_label('input', 1, 'u1')
      | port_label('output',1,'#ifdef u1');
      | port_label('output',2,'#else');
  bInterruptStep : Outport  RequirementInfo={} %GIDa_72cf4ec4_c922_4cb4_b7dc_ad31029b169c
  wires:
  Constant/1 -> Preprocessor IF/1
  u16BeltPayOutFiltered_mm/1 -> Belt Payout Abortion Opt Activated/3(u16BeltPayOutFiltered_mm)
  bBeltPayOutAbortion2/1 -> Belt Payout Abortion Opt Activated/1(bBeltPayOutAbortion2)
  Belt Payout Abortion Opt Deactivated/1(bShallStepContinue) -> Merge/1
  Belt Payout Abortion Opt Activated/1(bShallStepContinue) -> Merge/2
  Preprocessor IF/2 -> Belt Payout Abortion Opt Deactivated/Action
  Preprocessor IF/1 -> Belt Payout Abortion Opt Activated/Action
  Merge/1 -> bInterruptStep/1
  bBeltPayOutAbortion1/1 -> Belt Payout Abortion Opt Activated/2(bBeltPayOutAbortion1)

== system LIB_TF_G_12_StepControl/TF_G_12_ManageEndingStep/Step execution in progress/ManageMotorBlocked (Motor OverCurrent) ==
  u32MotorCurrent : Inport  RequirementInfo={} %GIDa_17936355_80b8_4cd3_b4c1_7db47cd26ca2
  u16Temperature : Inport  RequirementInfo={} %GIDa_61ba6760_456c_44f7_89b2_d2a7e55d2b0f  Port=2
  s16MotorPower : Inport  RequirementInfo={} %GIDa_b35d1c89_eab9_4b28_ad3c_9882880f1191  Port=3
  u16BatteryVoltage : Inport  RequirementInfo={} %GIDa_96467dde_b08f_45a8_b9c2_697b542d8526  Port=4
  bMotorBlockedControlled : Inport  RequirementInfo={} %GIDa_ec48f654_3f2a_47e8_a03b_effd5e2f0ea1  Port=5
  e_StepValidity Internal Status : Inport  RequirementInfo={} %GIDa_ec48f654_3f2a_47e8_a03b_effd5e2f0ea1  Port=6
  Constant2 : Constant  RequirementInfo={} %GIDa_3935372a_73bf_4c40_8c70_e63a57587ad8  SampleTime=-1  mask(TL_Constant){data={'output',{'variable','BFE_Config_PreProc/BFE_CFG_OPT_MOTOR_BLOCKED'},'date',735951.66847126163}}
      settings: CopyFcn=if exist('tl_reset_reviewflag','file')==2,tl_reset_reviewflag(gcbh);end  DeleteFcn=if exist('delete_tlblock','file')==2,delete_tlblock(gcbh);end  NameChangeFcn=if exist('rename_tlblock','file')==2,rename_tlblock(gcbh);end  OpenFcn=if exist('tl_open_blockdlg','file')==2,tl_open_blockdlg(gcbh);else,open_system(gcbh,'parameter');end
      mask Help: eval(['if exist(''tl_online_help'',''file'') == 2, tl_online_help(''Topic'',''TL_Constant''),else, web([''jar:file:///'',matlabroot,''/help/toolbox/simulink/help.jar!/slref/' lower(get_param(gcbh,'Blocktype')) '.html''], ''-helpbrowser''),end'])
      mask Display: plot([-0.05, 1.05, NaN, -0.05, 1.05],[.01, .01, NaN, .99, .99])
  Merge : Merge  Description=bTriggOffEvent :  RequirementInfo={} %GIDa_e75c5675_b191_4681_805b_71ff6cd2114b  InitialOutput=1  mask(TL_Merge){data={'comment',{'text',['bTriggOffEvent :']},'output',{'name','bMotorBlockedEvent'},'date',735951.66847087967}}
      settings: CopyFcn=if exist('tl_reset_reviewflag','file')==2,tl_reset_reviewflag(gcbh);end  DeleteFcn=if exist('delete_tlblock','file')==2,delete_tlblock(gcbh);end  NameChangeFcn=if exist('rename_tlblock','file')==2,rename_tlblock(gcbh);end  OpenFcn=if exist('tl_open_blockdlg','file')==2,tl_open_blockdlg(gcbh);else,open_system(gcbh,'parameter');end
      mask Help: eval(['if exist(''tl_online_help'',''file'') == 2, tl_online_help(''Topic'',''TL_Merge''),else, web([''jar:file:///'',matlabroot,''/help/toolbox/simulink/help.jar!/slref/' lower(get_param(gcbh,'Blocktype')) '.html''], ''-helpbrowser''),end'])
      mask Display: plot([-0.05, 1.05, NaN, -0.05, 1.05],[.01, .01, NaN, .99, .99])
  Motor Blocked Opt Activated : Subsystem  RequirementInfo={} %GIDa_52a70337_52e0_4369_bbd4_b5c5ccf0577c  TreatAsAtomicUnit=on
  Motor Blocked Opt Deactivated : Subsystem  RequirementInfo={} %GIDa_a82ba5df_7933_4cd3_bf8e_1b422b09be1a  TreatAsAtomicUnit=on
  Preprocessor IF : If  RequirementInfo={} %GIDa_4ce509fc_9768_4e92_9188_1690156df048  IfExpression=u1  mask(TL_PreProcessorIf){data={'mode',2,'date',735951.66845806711}}
      settings: DeleteFcn=if exist('delete_tlblock','file')==2,delete_tlblock(gcbh);end  NameChangeFcn=if exist('rename_tlblock','file')==2,rename_tlblock(gcbh);end  OpenFcn=if exist('tl_open_blockdlg','file')==2,tl_open_blockdlg(gcbh);else,open_system(gcbh,'parameter');end
      mask Help: eval(['if exist(''tl_online_help'',''file'') == 2, tl_online_help(''Topic'',''TL_PreProcessorIf''),else, web([''jar:file:///'',matlabroot,''/help/toolbox/simulink/help.jar!/slref/' lower(get_param(gcbh,'Blocktype')) '.html''], ''-helpbrowser''),end'])
      mask Display:
      | plot([-0.05, 1.05, NaN, -0.05, 1.05],[.01, .01, NaN, .99, .99])
      | 
      | port_label('input', 1, 'u1')
      | port_label('output',1,'#ifdef u1');
      | port_label('output',2,'#else');
  bInterruptStep : Outport  RequirementInfo={} %GIDa_48089b61_6961_4193_add9_901674722376
  wires:
  Motor Blocked Opt Activated/1(bInterruptStep) -> Merge/2
  Merge/1 -> bInterruptStep/1
  Constant2/1 -> Preprocessor IF/1
  Motor Blocked Opt Deactivated/1(bInterruptStep) -> Merge/1
  Preprocessor IF/2 -> Motor Blocked Opt Deactivated/Action
  Preprocessor IF/1 -> Motor Blocked Opt Activated/Action
  u32MotorCurrent/1 -> Motor Blocked Opt Activated/1(u32MotorCurrent)
  u16Temperature/1 -> Motor Blocked Opt Activated/2(u16Temperature)
  s16MotorPower/1 -> Motor Blocked Opt Activated/3(s16MotorPower)
  u16BatteryVoltage/1 -> Motor Blocked Opt Activated/4(u16BatteryVoltage)
  bMotorBlockedControlled/1 -> Motor Blocked Opt Activated/5(bMotorBlockedControlled)
  e_StepValidity Internal Status/1 -> Motor Blocked Opt Activated/6(e_StepValidity Internal Status)

== system LIB_TF_G_12_StepControl/TF_G_12_ManageEndingStep/Step execution in progress/ManageTriggOff (end of holding steps) ==
  bTriggOffControlled : Inport  RequirementInfo={} %GIDa_da2ae815_c72f_456c_b4c0_d787eb8f78c7
  bIsNoMoreTensioningSituation : Inport  RequirementInfo={} %GIDa_c845717b_516d_478e_aa10_74e6563548b3  Port=2
  Constant : Constant  RequirementInfo={} %GIDa_4b99f0d7_e827_4a9c_8cac_f57c76791725  SampleTime=-1  mask(TL_Constant){data={'output',{'variable','BFE_Config_PreProc/BFE_CFG_OPT_TRIGG_OFF'},'date',735951.6684578819}}
      settings: CopyFcn=if exist('tl_reset_reviewflag','file')==2,tl_reset_reviewflag(gcbh);end  DeleteFcn=if exist('delete_tlblock','file')==2,delete_tlblock(gcbh);end  NameChangeFcn=if exist('rename_tlblock','file')==2,rename_tlblock(gcbh);end  OpenFcn=if exist('tl_open_blockdlg','file')==2,tl_open_blockdlg(gcbh);else,open_system(gcbh,'parameter');end
      mask Help: eval(['if exist(''tl_online_help'',''file'') == 2, tl_online_help(''Topic'',''TL_Constant''),else, web([''jar:file:///'',matlabroot,''/help/toolbox/simulink/help.jar!/slref/' lower(get_param(gcbh,'Blocktype')) '.html''], ''-helpbrowser''),end'])
      mask Display: plot([-0.05, 1.05, NaN, -0.05, 1.05],[.01, .01, NaN, .99, .99])
  Merge : Merge  Description=bTriggOffEvent :  RequirementInfo={} %GIDa_f1a087dc_8221_4d34_806f_26988f073697  InitialOutput=1  mask(TL_Merge){data={'comment',{'text',['bTriggOffEvent :']},'output',{'name','bTriggOffEvent'},'date',735951.66845750005}}
      settings: CopyFcn=if exist('tl_reset_reviewflag','file')==2,tl_reset_reviewflag(gcbh);end  DeleteFcn=if exist('delete_tlblock','file')==2,delete_tlblock(gcbh);end  NameChangeFcn=if exist('rename_tlblock','file')==2,rename_tlblock(gcbh);end  OpenFcn=if exist('tl_open_blockdlg','file')==2,tl_open_blockdlg(gcbh);else,open_system(gcbh,'parameter');end
      mask Help: eval(['if exist(''tl_online_help'',''file'') == 2, tl_online_help(''Topic'',''TL_Merge''),else, web([''jar:file:///'',matlabroot,''/help/toolbox/simulink/help.jar!/slref/' lower(get_param(gcbh,'Blocktype')) '.html''], ''-helpbrowser''),end'])
      mask Display: plot([-0.05, 1.05, NaN, -0.05, 1.05],[.01, .01, NaN, .99, .99])
  Preprocessor IF : If  RequirementInfo={} %GIDa_fac5b1bb_0a70_44af_a03b_f02e28a18560  IfExpression=u1  mask(TL_PreProcessorIf){data={'mode',2,'date',735951.66845717595}}
      settings: DeleteFcn=if exist('delete_tlblock','file')==2,delete_tlblock(gcbh);end  NameChangeFcn=if exist('rename_tlblock','file')==2,rename_tlblock(gcbh);end  OpenFcn=if exist('tl_open_blockdlg','file')==2,tl_open_blockdlg(gcbh);else,open_system(gcbh,'parameter');end
      mask Help: eval(['if exist(''tl_online_help'',''file'') == 2, tl_online_help(''Topic'',''TL_PreProcessorIf''),else, web([''jar:file:///'',matlabroot,''/help/toolbox/simulink/help.jar!/slref/' lower(get_param(gcbh,'Blocktype')) '.html''], ''-helpbrowser''),end'])
      mask Display:
      | plot([-0.05, 1.05, NaN, -0.05, 1.05],[.01, .01, NaN, .99, .99])
      | 
      | port_label('input', 1, 'u1')
      | port_label('output',1,'#ifdef u1');
      | port_label('output',2,'#else');
  TriggOff Opt Activated : Subsystem  RequirementInfo={} %GIDa_0124550f_1351_46b6_85d9_d8e365461185  TreatAsAtomicUnit=on
  TriggOff Opt Deactivated : Subsystem  RequirementInfo={} %GIDa_e0c68771_cc2d_4ec0_9290_0bb86ee1a1e6  TreatAsAtomicUnit=on
  bInterruptStep : Outport  RequirementInfo={} %GIDa_441439b0_be7b_456e_837f_ab72d32e9697
  wires:
  Merge/1 -> bInterruptStep/1
  Preprocessor IF/1 -> TriggOff Opt Activated/Action
  Preprocessor IF/2 -> TriggOff Opt Deactivated/Action
  TriggOff Opt Activated/1(bInterruptStep) -> Merge/2
  TriggOff Opt Deactivated/1(bInterruptStep) -> Merge/1
  bTriggOffControlled/1 -> TriggOff Opt Activated/1(bTriggOffControlled)
  bIsNoMoreTensioningSituation/1 -> TriggOff Opt Activated/2(bIsNoMoreTensioningSituation)
  Constant/1 -> Preprocessor IF/1

== system LIB_TF_G_12_StepControl/TF_G_12_ControlStepExecution/New Step started/Adapt Step Target Value/No Temperature Adaptation ==
  Action Port : ActionPort
  KU8_NO_WEIGHT : Constant  RequirementInfo={} %GIDa_cbf50fb2_205d_4e2b_b435_8e11c0676f9a  Value=ddv('BFE/KUC_NEUTRAL_WEIGHT')  OutDataTypeStr=uint8  mask(TL_Constant){data={'output',{'variable','BFE/KUC_NEUTRAL_WEIGHT'},'date',735951.66799453704}}
      settings: CopyFcn=if exist('tl_reset_reviewflag','file')==2,tl_reset_reviewflag(gcbh);end  DeleteFcn=if exist('delete_tlblock','file')==2,delete_tlblock(gcbh);end  NameChangeFcn=if exist('rename_tlblock','file')==2,rename_tlblock(gcbh);end  OpenFcn=if exist('tl_open_blockdlg','file')==2,tl_open_blockdlg(gcbh);else,open_system(gcbh,'parameter');end
      mask Help: eval(['if exist(''tl_online_help'',''file'') == 2, tl_online_help(''Topic'',''TL_Constant''),else, web([''jar:file:///'',matlabroot,''/help/toolbox/simulink/help.jar!/slref/' lower(get_param(gcbh,'Blocktype')) '.html''], ''-helpbrowser''),end'])
      mask Display: plot([-0.05, 1.05, NaN, -0.05, 1.05],[.01, .01, NaN, .99, .99])
  Out1 : Outport  InitialOutput=64
  wires:
  KU8_NO_WEIGHT/1 -> Out1/1
